simulink model "lecture03c_pendulum_example_model"  (Simulink 9.2)
settings: Solver=ode45  StartTime=0.0  StopTime=10.0  MaxStep=dtMax  RelTol=1e-3  EnableMultiTasking=on
undefined symbols (not defined in the file): b, g, L, m, theta0, thetaDot0
settings Model: Creator=lumch  LastModifiedBy=Christopher
settings OptimizationCC: ExpressionDepthLimit=2147483647
settings DebuggingCC: SolverPrmCheckMsg=warning

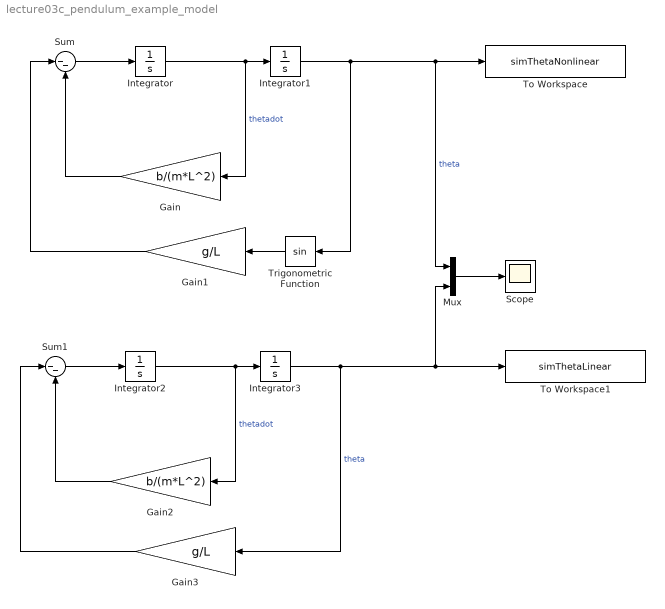
== system lecture03c_pendulum_example_model ==
  Gain : Gain  Gain=b/(m*L^2)
  Gain1 : Gain  Gain=g/L
  Gain2 : Gain  Gain=b/(m*L^2)
  Gain3 : Gain  Gain=g/L
  Integrator : Integrator  InitialCondition=thetaDot0
  Integrator1 : Integrator  InitialCondition=theta0
  Integrator2 : Integrator  InitialCondition=thetaDot0
  Integrator3 : Integrator  InitialCondition=theta0
  Mux : Mux  Inputs=2
  Scope : Scope
  Sum : Sum  Inputs=|--
  Sum1 : Sum  Inputs=|--
  To Workspace : ToWorkspace  VariableName=simThetaNonlinear  SaveFormat=Structure With Time  SampleTime=-1
  To Workspace1 : ToWorkspace  VariableName=simThetaLinear  SaveFormat=Structure With Time  SampleTime=-1
  Trigonometric Function : Trigonometry
  wires:
  Integrator/1 -> Integrator1/1, Gain/1  "thetadot"
  Integrator1/1 -> Trigonometric Function/1, Mux/1, To Workspace/1  "theta"
  Gain/1 -> Sum/2
  Sum/1 -> Integrator/1
  Trigonometric Function/1 -> Gain1/1
  Gain1/1 -> Sum/1
  Integrator2/1 -> Integrator3/1, Gain2/1  "thetadot"
  Integrator3/1 -> Gain3/1, Mux/2, To Workspace1/1  "theta"
  Gain2/1 -> Sum1/2
  Sum1/1 -> Integrator2/1
  Gain3/1 -> Sum1/1
  Mux/1 -> Scope/1
